simulink model "LqrSpeedTest1_17a"  (R2017a)
settings: Solver=VariableStepAuto  StartTime=0.0  StopTime=15  RelTol=1e-3
values from neighbouring files (symbols this model uses):
  A = Gss.A    [TFfinder.m]
  B = Gss.B    [TFfinder.m]
  C = tf(PID*Gm)    [PIDtest1.m]    (also in TFfinder.m = Gss.C)
settings Model: Creator=Yahya  LastModifiedBy=Yahya

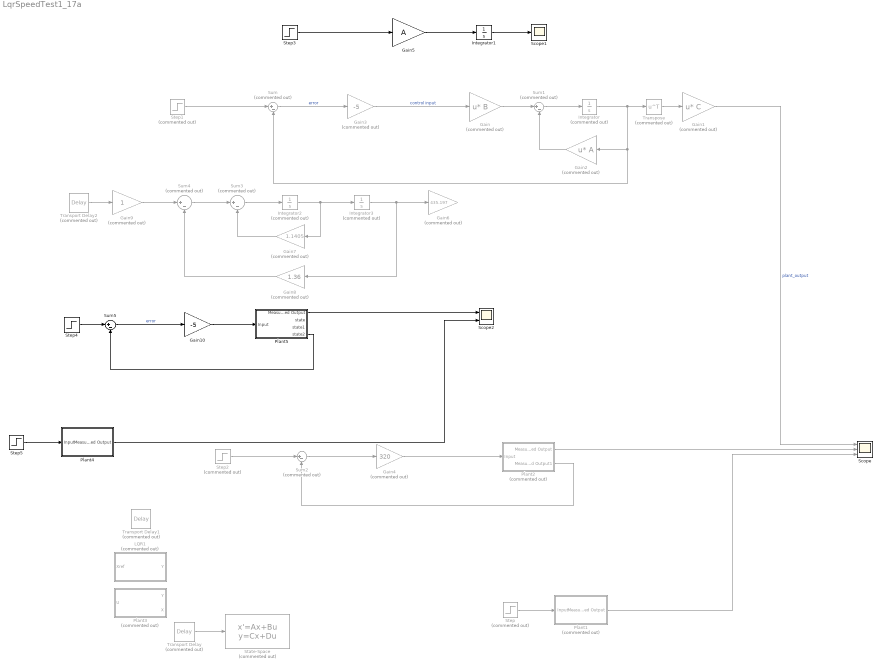
== system LqrSpeedTest1_17a ==
  Gain : Gain  Commented=on  Gain=B  Multiplication=Matrix(u*K)
  Gain1 : Gain  Commented=on  Gain=C  Multiplication=Matrix(u*K)
  Gain10 : Gain  Gain=-5
  Gain2 : Gain  Commented=on  Gain=A  Multiplication=Matrix(u*K)
  Gain3 : Gain  Commented=on  Gain=-5
  Gain4 : Gain  Commented=on  Gain=320
  Gain5 : Gain  Gain=A
  Gain6 : Gain  Commented=on  Gain=435.197
  Gain7 : Gain  Commented=on  Gain=1.1405
  Gain8 : Gain  Commented=on  Gain=1.36
  Gain9 : Gain  Commented=on
  Integrator : Integrator  Commented=on
  Integrator1 : Integrator
  Integrator2 : Integrator  Commented=on
  Integrator3 : Integrator  Commented=on
  LQR1 : Subsystem  Commented=on
  Plant1 : Subsystem  Commented=on
  Plant2 : Subsystem  Commented=on
  Plant3 : Subsystem  Commented=on
  Plant4 : Subsystem
  Plant5 : Subsystem
  Scope : Scope  NumInputPorts=3
  Scope1 : Scope
  Scope2 : Scope  NumInputPorts=2
  State-Space : StateSpace  Commented=on  A=A  B=B  C=C  D=0  X0=0
  Step : Step  Commented=on  SampleTime=0
  Step1 : Step  Commented=on  SampleTime=0
  Step2 : Step  Commented=on  SampleTime=0
  Step3 : Step  SampleTime=0
  Step4 : Step  SampleTime=0
  Step5 : Step  SampleTime=0
  Sum{,1..4} (5 alike) : Sum  Commented=on  Inputs=|+-
  Sum5 : Sum  Inputs=|+-
  Transport Delay : TransportDelay  Commented=on  DelayTime=0.3
  Transport Delay1 : TransportDelay  Commented=on  DelayTime=0.3
  Transport Delay2 : TransportDelay  Commented=on  DelayTime=0.3
  Transpose : Math  Commented=on  Operator=transpose  SaturateOnIntegerOverflow=on
  wires:
  Sum/1 -> Gain3/1  "error"
  Step/1 -> Plant1/1(Input)
  Integrator/1 -> Transpose/1, Gain2/1, Sum/2
  Gain1/1 -> Scope/1  "plant_output"
  Sum1/1 -> Integrator/1
  Gain2/1 -> Sum1/2
  Gain/1 -> Sum1/1
  Gain3/1 -> Gain/1  "control input"
  Step1/1 -> Sum/1
  Transpose/1 -> Gain1/1
  Gain4/1 -> Plant2/1(Input)
  Plant1/1(Measured Output) -> Scope/3
  Transport Delay/1 -> State-Space/1
  Plant2/1(Measured Output) -> Scope/2
  Step2/1 -> Sum2/1
  Sum2/1 -> Gain4/1
  Plant2/2(Measured Output1) -> Sum2/2
  Gain5/1 -> Integrator1/1
  Step3/1 -> Gain5/1
  Integrator1/1 -> Scope1/1
  Sum3/1 -> Integrator2/1
  Integrator2/1 -> Gain7/1, Integrator3/1
  Integrator3/1 -> Gain8/1, Gain6/1
  Sum4/1 -> Sum3/1
  Gain7/1 -> Sum3/2
  Gain8/1 -> Sum4/2
  Gain9/1 -> Sum4/1
  Step5/1 -> Plant4/1(Input)
  Plant4/1(Measured Output) -> Scope2/2
  Transport Delay2/1 -> Gain9/1
  Plant5/1(Measured Output) -> Scope2/1
  Sum5/1 -> Gain10/1  "error"
  Step4/1 -> Sum5/1
  Gain10/1 -> Plant5/1(Input)
  Plant5/4(state2) -> Sum5/2

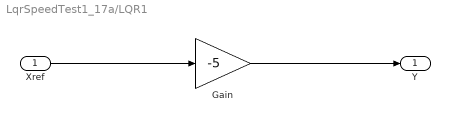
== system LqrSpeedTest1_17a/LQR1 ==
  Xref : Inport
  Gain : Gain  Gain=-5
  Y : Outport
  wires:
  Xref/1 -> Gain/1
  Gain/1 -> Y/1

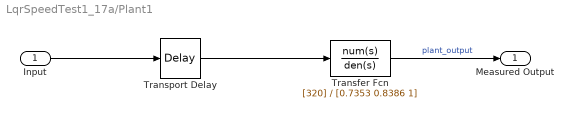
== system LqrSpeedTest1_17a/Plant1 ==
  Input : Inport
  Transfer Fcn : TransferFcn  Numerator=[320]  Denominator=[0.7353 0.8386 1]
  Transport Delay : TransportDelay  DelayTime=0.3
  Measured Output : Outport
  wires:
  Input/1 -> Transport Delay/1
  Transfer Fcn/1 -> Measured Output/1  "plant_output"
  Transport Delay/1 -> Transfer Fcn/1

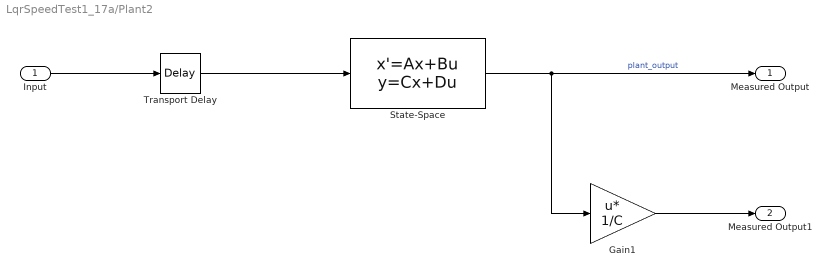
== system LqrSpeedTest1_17a/Plant2 ==
  Input : Inport
  Gain1 : Gain  Gain=1/C  Multiplication=Matrix(u*K)
  State-Space : StateSpace  A=A  B=B  C=C  D=0  X0=0
  Transport Delay : TransportDelay  DelayTime=0.3
  Measured Output : Outport
  Measured Output1 : Outport  Port=2
  wires:
  Input/1 -> Transport Delay/1
  State-Space/1 -> Gain1/1, Measured Output/1  "plant_output"
  Transport Delay/1 -> State-Space/1
  Gain1/1 -> Measured Output1/1

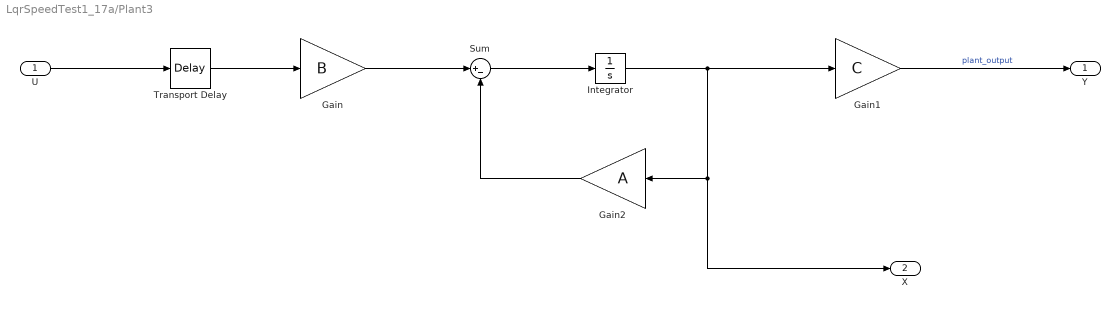
== system LqrSpeedTest1_17a/Plant3 ==
  U : Inport
  Gain : Gain  Gain=B
  Gain1 : Gain  Gain=C
  Gain2 : Gain  Gain=A
  Integrator : Integrator
  Sum : Sum  Inputs=|+-
  Transport Delay : TransportDelay  DelayTime=0.3
  Y : Outport
  X : Outport  Port=2
  wires:
  U/1 -> Transport Delay/1
  Gain1/1 -> Y/1  "plant_output"
  Sum/1 -> Integrator/1
  Gain/1 -> Sum/1
  Integrator/1 -> Gain2/1, X/1, Gain1/1
  Gain2/1 -> Sum/2
  Transport Delay/1 -> Gain/1

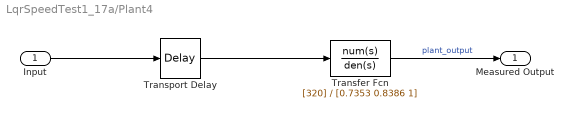
== system LqrSpeedTest1_17a/Plant4 ==
  Input : Inport
  Transfer Fcn : TransferFcn  Numerator=[320]  Denominator=[0.7353 0.8386 1]
  Transport Delay : TransportDelay  DelayTime=0.3
  Measured Output : Outport
  wires:
  Input/1 -> Transport Delay/1
  Transfer Fcn/1 -> Measured Output/1  "plant_output"
  Transport Delay/1 -> Transfer Fcn/1

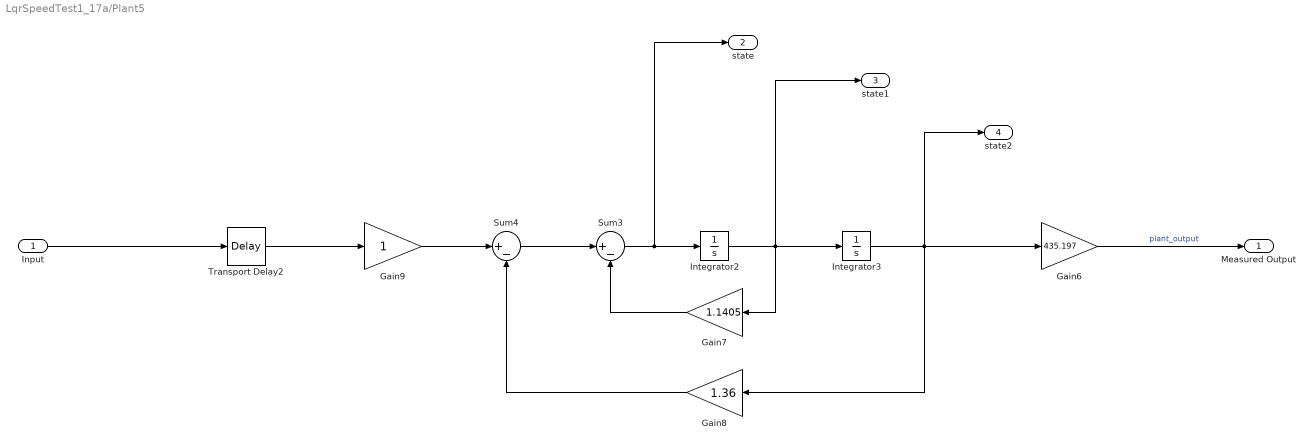
== system LqrSpeedTest1_17a/Plant5 ==
  Input : Inport
  Gain6 : Gain  Gain=435.197
  Gain7 : Gain  Gain=1.1405
  Gain8 : Gain  Gain=1.36
  Gain9 : Gain
  Integrator2 : Integrator
  Integrator3 : Integrator
  Sum3 : Sum  Inputs=|+-
  Sum4 : Sum  Inputs=|+-
  Transport Delay2 : TransportDelay  DelayTime=0.3
  Measured Output : Outport
  state : Outport  Port=2
  state1 : Outport  Port=3
  state2 : Outport  Port=4
  wires:
  Gain6/1 -> Measured Output/1  "plant_output"
  Gain7/1 -> Sum3/2
  Transport Delay2/1 -> Gain9/1
  Integrator3/1 -> state2/1, Gain8/1, Gain6/1
  Gain8/1 -> Sum4/2
  Sum3/1 -> state/1, Integrator2/1
  Sum4/1 -> Sum3/1
  Input/1 -> Transport Delay2/1
  Integrator2/1 -> state1/1, Gain7/1, Integrator3/1
  Gain9/1 -> Sum4/1
